simulink model "modelo_2"  (R2023a)
settings: Solver=VariableStepAuto  StartTime=0.0  StopTime=100  RelTol=1e-3
InitFcn:
  | parametros
  | gain_CL
values from neighbouring files (symbols this model uses):
  b_ha = (n_h*w_des_h+2*dseta_h*w_des_h)*(J_hEq)-b_hEq    [gain_CL.m]
  b_hd = 8    [parametros.m]
  b_hm = 18    [parametros.m]
  b_t = 90    [parametros.m]
  b_ta = (n_t*w_des_t+2*dseta_t*w_des_t)*(J_tEq)-b_tEq    [gain_CL.m]
  b_td = 1.8    [parametros.m]
  b_tm = 6    [parametros.m]
  i_h = 22    [parametros.m]
  i_t = 30    [parametros.m]
  J_hd_hEb = 3800    [parametros.m]
  J_hm_hb = 30    [parametros.m]
  J_td = 1200    [parametros.m]
  J_tm_tb = 7    [parametros.m]
  k_hsa = (w_des_h^2+2*dseta_h*w_des_h)*(J_hEq)    [gain_CL.m]
  k_hsia = (w_des_h^3)*(J_hEq)    [gain_CL.m]
  k_tsa = (w_des_t^2+2*dseta_t*w_des_t)*(J_tEq)    [gain_CL.m]
  k_tsia = (w_des_t^3)*(J_tEq)    [gain_CL.m]
  m_l = M_s    (= 15000)    [parametros.m]    (also in polos_inclinacion.m = M_s)
  M_t = 30000    [parametros.m]
  r_hd = 0.75    [parametros.m]
  r_td = 0.50    (= 0.5)    [parametros.m]
  T_s = (b_hEq/J_hEq)/2/pi/100    (= 0.000679331161018)    [parametros.m]
libraries: simulink x8
settings Model: Creator=Usuario  LastModifiedBy=Usuario

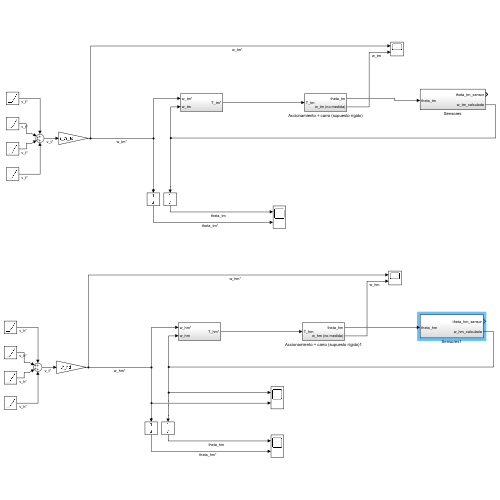
[thumbnail: Simulink's stored preview of the top-level diagram]
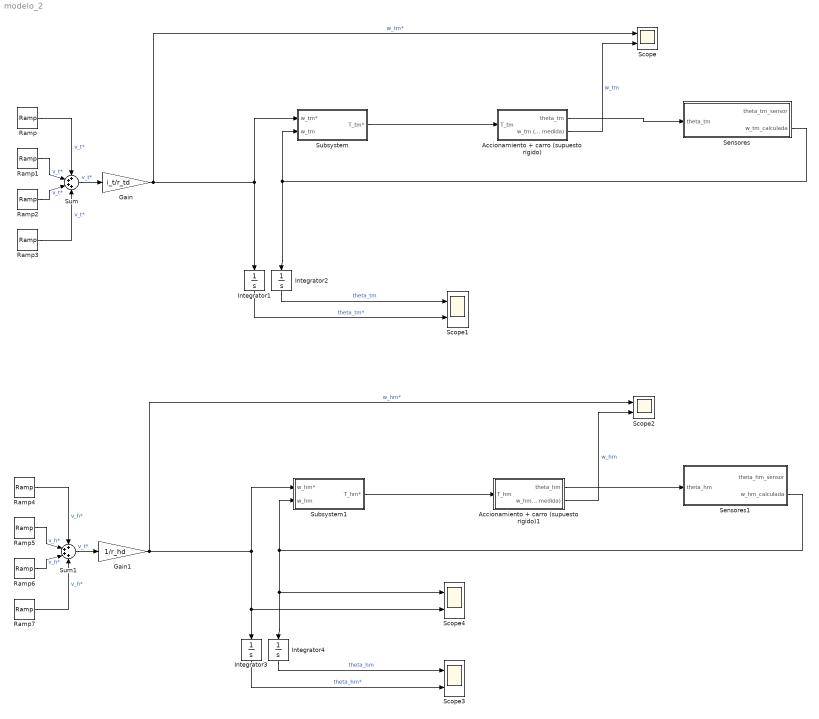
== system modelo_2 ==
  Accionamiento + carro (supuesto rígido) : Subsystem
  Accionamiento + carro (supuesto rígido)1 : Subsystem
  Gain : Gain  Gain=i_t/r_td
  Gain1 : Gain  Gain=1/r_hd
  Integrator{1..4} (4 alike) : Integrator
  Ramp : simulink/Sources/Ramp  slope=0.8  start=5  InitialOutput=0
  Ramp1 : simulink/Sources/Ramp  slope=-0.8  start=10  InitialOutput=0
  Ramp2 : simulink/Sources/Ramp  slope=-0.8  start=35  InitialOutput=0
  Ramp3 : simulink/Sources/Ramp  slope=0.8  start=40  InitialOutput=0
  Ramp4 : simulink/Sources/Ramp  slope=0.8  start=5  InitialOutput=0
  Ramp5 : simulink/Sources/Ramp  slope=-0.8  start=10  InitialOutput=0
  Ramp6 : simulink/Sources/Ramp  slope=-0.8  start=35  InitialOutput=0
  Ramp7 : simulink/Sources/Ramp  slope=0.8  start=40  InitialOutput=0
  Scope{,1..4} (5 alike) : Scope  NumInputPorts=2
  Sensores : Subsystem
  Sensores1 : Subsystem
  Subsystem : Subsystem
  Subsystem1 : Subsystem
  Sum : Sum  Inputs=++++
  Sum1 : Sum  Inputs=++++
  wires:
  Subsystem/1(T_tm*) -> Accionamiento + carro (supuesto rígido)/1(T_tm)
  Ramp/1 -> Sum/1  "v_t*"
  Ramp2/1 -> Sum/3  "v_t*"
  Ramp3/1 -> Sum/4  "v_t*"
  Ramp1/1 -> Sum/2  "v_t*"
  Sum/1 -> Gain/1  "v_t*"
  Integrator1/1 -> Scope1/2  "theta_tm*"
  Integrator2/1 -> Scope1/1  "theta_tm"
  Accionamiento + carro (supuesto rígido)/1(theta_tm) -> Sensores/1(theta_tm)
  Gain/1 -> Subsystem/1(w_tm*), Integrator1/1, Scope/1  "w_tm*"
  Accionamiento + carro (supuesto rígido)/2(w_tm (no medida)) -> Scope/2  "w_tm"
  Sensores/2(w_tm_calculada) -> Integrator2/1, Subsystem/2(w_tm)
  Subsystem1/1(T_hm*) -> Accionamiento + carro (supuesto rígido)1/1(T_hm)
  Ramp5/1 -> Sum1/2  "v_h*"
  Gain1/1 -> Subsystem1/1(w_hm*), Scope4/2, Integrator3/1, Scope2/1  "w_hm*"
  Ramp6/1 -> Sum1/3  "v_h*"
  Sum1/1 -> Gain1/1  "v_t*"
  Accionamiento + carro (supuesto rígido)1/2(w_hm (no medida)) -> Scope2/2  "w_hm"
  Accionamiento + carro (supuesto rígido)1/1(theta_hm) -> Sensores1/1(theta_hm)
  Sensores1/2(w_hm_calculada) -> Scope4/1, Integrator4/1, Subsystem1/2(w_hm)
  Ramp4/1 -> Sum1/1  "v_h*"
  Integrator3/1 -> Scope3/2  "theta_hm*"
  Integrator4/1 -> Scope3/1  "theta_hm"
  Ramp7/1 -> Sum1/4  "v_h*"

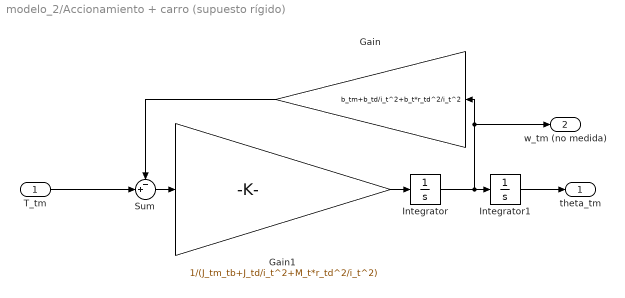
== system modelo_2/Accionamiento + carro (supuesto rígido) ==
  T_tm : Inport
  Gain : Gain  Gain=b_tm+b_td/i_t^2+b_t*r_td^2/i_t^2
  Gain1 : Gain  Gain=1/(J_tm_tb+J_td/i_t^2+M_t*r_td^2/i_t^2)
  Integrator : Integrator
  Integrator1 : Integrator
  Sum : Sum  Inputs=-+|
  theta_tm : Outport
  w_tm (no medida) : Outport  Port=2
  wires:
  Integrator1/1 -> theta_tm/1
  T_tm/1 -> Sum/2
  Gain/1 -> Sum/1
  Sum/1 -> Gain1/1
  Gain1/1 -> Integrator/1
  Integrator/1 -> w_tm (no medida)/1, Gain/1, Integrator1/1

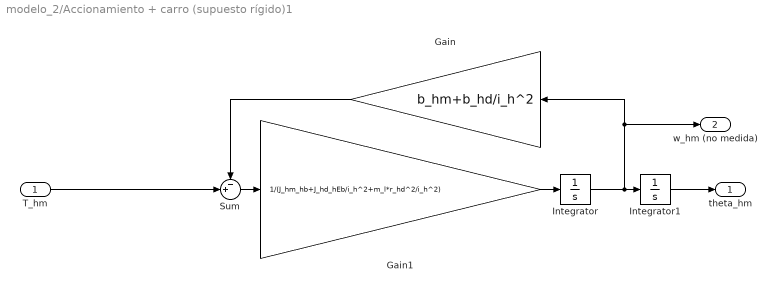
== system modelo_2/Accionamiento + carro (supuesto rígido)1 ==
  T_hm : Inport
  Gain : Gain  Gain=b_hm+b_hd/i_h^2
  Gain1 : Gain  Gain=1/(J_hm_hb+J_hd_hEb/i_h^2+m_l*r_hd^2/i_h^2)
  Integrator : Integrator
  Integrator1 : Integrator
  Sum : Sum  Inputs=-+|
  theta_hm : Outport
  w_hm (no medida) : Outport  Port=2
  wires:
  Integrator1/1 -> theta_hm/1
  T_hm/1 -> Sum/2
  Gain/1 -> Sum/1
  Sum/1 -> Gain1/1
  Gain1/1 -> Integrator/1
  Integrator/1 -> w_hm (no medida)/1, Gain/1, Integrator1/1

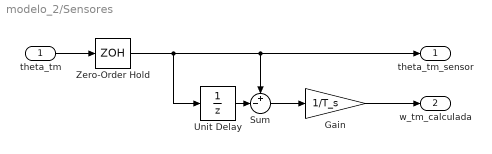
== system modelo_2/Sensores ==
  theta_tm : Inport
  Gain : Gain  Gain=1/T_s
  Sum : Sum  Inputs=+-|
  Unit Delay : UnitDelay  SampleTime=-1  HasFrameUpgradeWarning=on
  Zero-Order Hold : ZeroOrderHold  SampleTime=T_s
  theta_tm_sensor : Outport
  w_tm_calculada : Outport  Port=2
  wires:
  theta_tm/1 -> Zero-Order Hold/1
  Zero-Order Hold/1 -> Unit Delay/1, Sum/1, theta_tm_sensor/1
  Unit Delay/1 -> Sum/2
  Sum/1 -> Gain/1
  Gain/1 -> w_tm_calculada/1

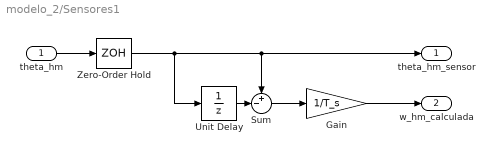
== system modelo_2/Sensores1 ==
  theta_hm : Inport
  Gain : Gain  Gain=1/T_s
  Sum : Sum  Inputs=+-|
  Unit Delay : UnitDelay  SampleTime=-1  HasFrameUpgradeWarning=on
  Zero-Order Hold : ZeroOrderHold  SampleTime=T_s
  theta_hm_sensor : Outport
  w_hm_calculada : Outport  Port=2
  wires:
  theta_hm/1 -> Zero-Order Hold/1
  Zero-Order Hold/1 -> Unit Delay/1, Sum/1, theta_hm_sensor/1
  Unit Delay/1 -> Sum/2
  Sum/1 -> Gain/1
  Gain/1 -> w_hm_calculada/1

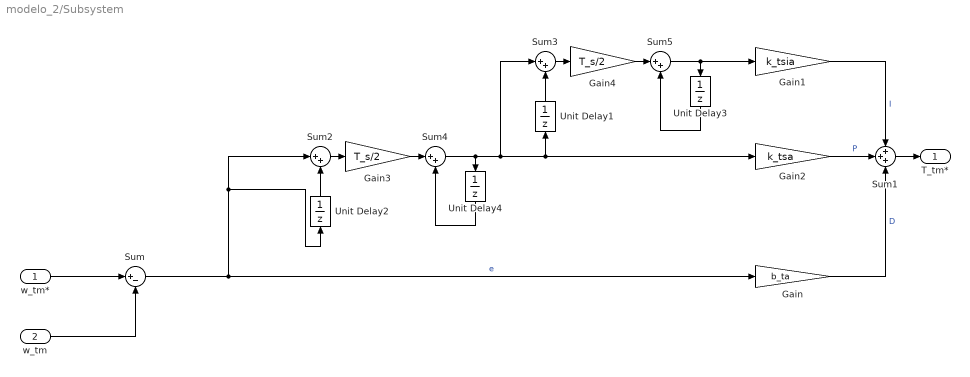
== system modelo_2/Subsystem ==
  w_tm* : Inport
  w_tm : Inport  Port=2
  Gain : Gain  Gain=b_ta
  Gain1 : Gain  Gain=k_tsia
  Gain2 : Gain  Gain=k_tsa
  Gain3 : Gain  Gain=T_s/2
  Gain4 : Gain  Gain=T_s/2
  Sum : Sum  Inputs=|+-
  Sum1 : Sum  Inputs=+++
  Sum{2..5} (4 alike) : Sum  Inputs=|++
  Unit Delay{1..4} (4 alike) : UnitDelay  SampleTime=-1  HasFrameUpgradeWarning=on
  T_tm* : Outport
  wires:
  Gain2/1 -> Sum1/2  "P"
  w_tm*/1 -> Sum/1
  Gain/1 -> Sum1/3  "D"
  Gain1/1 -> Sum1/1  "I"
  w_tm/1 -> Sum/2
  Sum1/1 -> T_tm*/1
  Unit Delay1/1 -> Sum3/2
  Sum3/1 -> Gain4/1
  Sum5/1 -> Gain1/1, Unit Delay3/1
  Unit Delay3/1 -> Sum5/2
  Gain4/1 -> Sum5/1
  Sum4/1 -> Sum3/1, Unit Delay1/1, Gain2/1, Unit Delay4/1
  Unit Delay4/1 -> Sum4/2
  Gain3/1 -> Sum4/1
  Unit Delay2/1 -> Sum2/2
  Sum2/1 -> Gain3/1
  Sum/1 -> Unit Delay2/1, Sum2/1, Gain/1  "e"

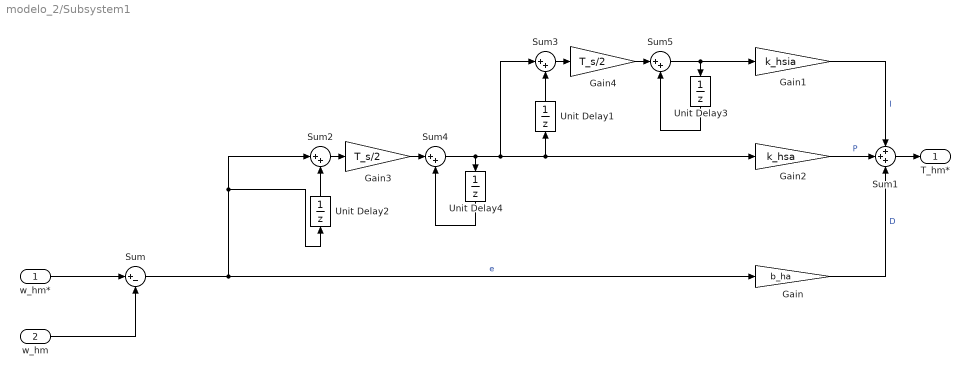
== system modelo_2/Subsystem1 ==
  w_hm* : Inport
  w_hm : Inport  Port=2
  Gain : Gain  Gain=b_ha
  Gain1 : Gain  Gain=k_hsia
  Gain2 : Gain  Gain=k_hsa
  Gain3 : Gain  Gain=T_s/2
  Gain4 : Gain  Gain=T_s/2
  Sum : Sum  Inputs=|+-
  Sum1 : Sum  Inputs=+++
  Sum{2..5} (4 alike) : Sum  Inputs=|++
  Unit Delay{1..4} (4 alike) : UnitDelay  SampleTime=-1  HasFrameUpgradeWarning=on
  T_hm* : Outport
  wires:
  Gain2/1 -> Sum1/2  "P"
  w_hm*/1 -> Sum/1
  Gain/1 -> Sum1/3  "D"
  Gain1/1 -> Sum1/1  "I"
  w_hm/1 -> Sum/2
  Sum1/1 -> T_hm*/1
  Unit Delay1/1 -> Sum3/2
  Sum3/1 -> Gain4/1
  Sum5/1 -> Gain1/1, Unit Delay3/1
  Unit Delay3/1 -> Sum5/2
  Gain4/1 -> Sum5/1
  Sum4/1 -> Sum3/1, Unit Delay1/1, Gain2/1, Unit Delay4/1
  Unit Delay4/1 -> Sum4/2
  Gain3/1 -> Sum4/1
  Unit Delay2/1 -> Sum2/2
  Sum2/1 -> Gain3/1
  Sum/1 -> Unit Delay2/1, Sum2/1, Gain/1  "e"
